simulink model "sampleModel2061"  (R2023a)
settings: Solver=VariableStepAuto  StartTime=0.0  StopTime=10.0  RelTol=1e-3
libraries: hdlsllib x5
settings Model: Creator=user1  LastModifiedBy=user1

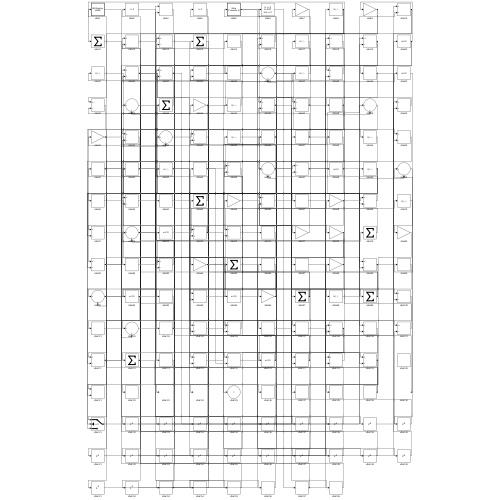
[thumbnail: Simulink's stored preview of the top-level diagram]
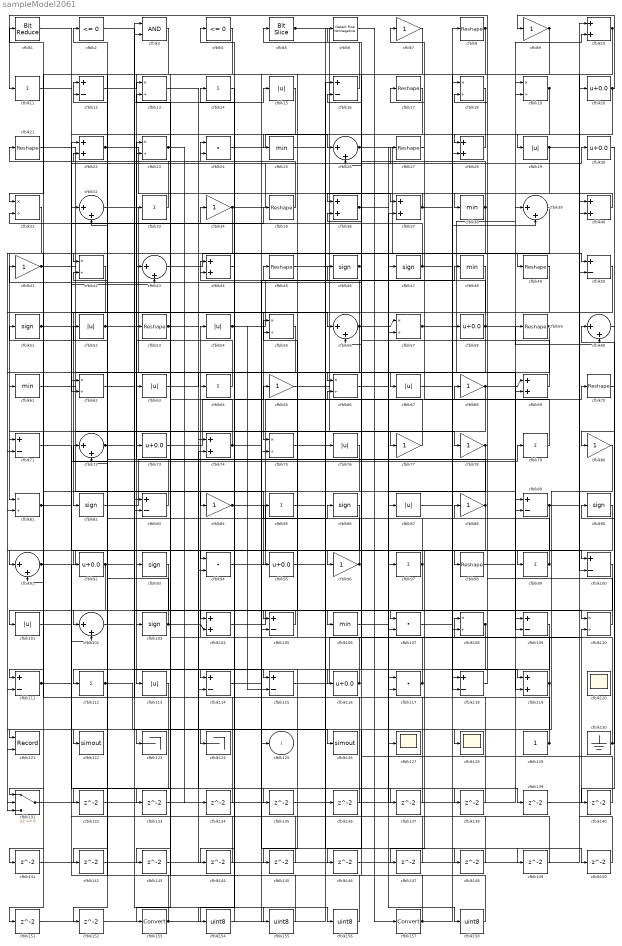
== system sampleModel2061 ==
  cfblk1 : hdlsllib/Logic and Bit Operations/Bit Reduce  mode=AND
  cfblk{10,22,28,36..37,40,44,69,74,104,119} (11 alike) : Sum
  cfblk{12,16,50,71,83,89,100,105,109,111,114..115,118} (13 alike) : Sum  Inputs=+-
  cfblk{15,29,52,54,63,67,76,87,101,113} (10 alike) : Abs  SaturateOnIntegerOverflow=off
  cfblk{26,32,39,43,56,60,72,91,102} (9 alike) : Sum  Inputs=|++
  cfblk{46..47,51,82,86,90,93,103} (8 alike) : Signum
  cfblk{25,38,48,61,106} (5 alike) : MinMax
  cfblk{24,94,107,117} (4 alike) : DotProduct  OutDataTypeStr=Inherit: Inherit via internal rule
  cfblk{13,18..19,23,31,42,55,57,62,66,75,81,108,110} (14 alike) : Product  Inputs=*/  RndMeth=Zero  SaturateOnIntegerOverflow=on
  cfblk{11,14,33,64,79,85,97,99,112} (9 alike) : Sum  Inputs=+
  cfblk{20,30,58,73,92,95,116} (7 alike) : Bias  Bias=0.0  SaturateOnIntegerOverflow=off
  cfblk120 : Scope
      settings: Floating=on
  cfblk121 : Record  FileSettingsInternal="{\"entries\":[{\"content\":{\"excelSettings\":{\"content\":{},\"type\":\"Streamout.ExcelSettings\"}},\"type\":\"Streamout.FileSettingStorage\",\"uuid\":\"\"}],\"packageUris\":[\"http:\\/\\/schema.mathworks.com\\/mf0\\/streamout_blocks\\/R2020a\"],\"version\":\"1.0\"}"  Layout=[1 1]  SignalsInternal="{\"entries\":[{\"content\":{\"signals\":[{\"content\":{\"blockPath\":[],\"dimensions\":[1],\"domain\":\"\",\"lineColor\":\"#a2142f\",\"plots\":[1],\"port\":1,\"signalID\":6369,\"signalName\":\"XY Graph:1\"},\"type\":\"RecordBlkView.Signal\",\"uuid\":\"\"},{\"content\":{\"blockPath\":[],\"dimensions\":[1],\"domain\":\"\",\"lineColor\":\"#139fff\",\"plots\":[1],\"port\":2,\"signalID\":6372,\"signalName\":\"XY Graph:2\"},\"type\":\"RecordBlkView.Signal\",\"uuid\":\"\"}]},\"type\":\"RecordBlkView.InputSignals\",\"uuid\":\"\"}],\"packageUris\":[\"http:\\/\\/schema.mathworks.com\\/mf0\\/streamout_blocks\\/R2020a\"],\"version\":\"1.0\"}"  VisualizationBindings="{\"xyplotplugin\":{\"info\":[{\"series\":[{\"bindingParametersList\":[{\"parameter\":\"X-Axis\",\"signalID\":6369,\"signalName\":\"XY Graph:1\"},{\"parameter\":\"Y-Axis\",\"signalID\":6372,\"signalName\":\"XY Graph:2\"}],\"seriesID\":44512}],\"subplotID\":1}]}}"  CompatibilityTag=XY  st=-1
  cfblk122 : ToWorkspace  VariableName=simout  SaveFormat=Timeseries  SampleTime=-1
  cfblk123 : Terminator
  cfblk124 : Terminator
  cfblk126 : ToWorkspace  VariableName=simout  SaveFormat=Timeseries  SampleTime=-1
  cfblk127 : Scope
  cfblk128 : Scope
  cfblk129 : Constant  SampleTime=-1
  cfblk130 : Ground
  cfblk131 : Switch  SaturateOnIntegerOverflow=off  InputSameDT=off
  cfblk{132..152} (21 alike) : Delay  SampleTime=1
  cfblk153 : DataTypeConversion  SaturateOnIntegerOverflow=off  RndMeth=Floor
  cfblk{154..156,158} (4 alike) : DataTypeConversion  OutDataTypeStr=uint8  SaturateOnIntegerOverflow=off  RndMeth=Floor
  cfblk157 : DataTypeConversion  SaturateOnIntegerOverflow=off  RndMeth=Floor
  cfblk{8,17,21,27,35,45,49,53,59,70,98} (11 alike) : Reshape
  cfblk2 : hdlsllib/Logic and Bit Operations/Compare To Zero  relop=<=  OutDataTypeStr=boolean
  cfblk3 : Logic  AllPortsSameDT=off  OutDataTypeStr=boolean
  cfblk{7,9,34,41,65,68,77..78,80,84,88,96} (12 alike) : Gain
  cfblk4 : hdlsllib/Logic and Bit Operations/Compare To Zero  relop=<=  OutDataTypeStr=boolean
  cfblk5 : hdlsllib/Logic and Bit Operations/Bit Slice  lidx=7  ridx=0
  cfblk6 : hdlsllib/Logic and Bit Operations/Detect Rise Nonnegative  vinit=0  OutDataTypeStr=boolean
  cfblk125 : Outport  VectorParamsAs1DForOutWhenUnconnected=off
  wires:
  cfblk76/1 -> cfblk113/1
  cfblk31/1 -> cfblk81/1
  cfblk8/1 -> cfblk103/1, cfblk105/1, cfblk105/2
  cfblk99/1 -> cfblk11/1, cfblk12/2
  cfblk5/1 -> cfblk77/1, cfblk148/1
  cfblk24/1 -> cfblk26/1
  cfblk42/1 -> cfblk82/1
  cfblk80/1 -> cfblk128/1
  cfblk94/1 -> cfblk70/1
  cfblk83/1 -> cfblk23/1
  cfblk17/1 -> cfblk102/1
  cfblk36/1 -> cfblk106/1, cfblk158/1
  cfblk81/1 -> cfblk79/1, cfblk35/1
  cfblk119/1 -> cfblk108/1, cfblk131/2, cfblk146/1
  cfblk116/1 -> cfblk54/1, cfblk43/1
  cfblk55/1 -> cfblk111/1
  cfblk56/1 -> cfblk57/1, cfblk14/1, cfblk100/1, cfblk91/2
  cfblk60/1 -> cfblk90/1
  cfblk58/1 -> cfblk45/1, cfblk60/2, cfblk71/2
  cfblk130/1 -> cfblk24/1, cfblk60/1
  cfblk6/1 -> cfblk157/1
  cfblk91/1 -> cfblk98/1, cfblk102/2
  cfblk15/1 -> cfblk63/1
  cfblk87/1 -> cfblk108/2
  cfblk79/1 -> cfblk17/1
  cfblk53/1 -> cfblk115/1, cfblk109/2
  cfblk49/1 -> cfblk101/1
  cfblk40/1 -> cfblk38/1
  cfblk78/1 -> cfblk141/1, cfblk142/1
  cfblk75/1 -> cfblk68/1
  cfblk52/1 -> cfblk109/1, cfblk114/2
  cfblk46/1 -> cfblk96/1, cfblk26/2
  cfblk21/1 -> cfblk95/1
  cfblk16/1 -> cfblk5/1
  cfblk112/1 -> cfblk126/1, cfblk12/1
  cfblk118/1 -> cfblk18/2
  cfblk32/1 -> cfblk89/1
  cfblk96/1 -> cfblk24/2, cfblk66/2
  cfblk27/1 -> cfblk7/1
  cfblk45/1 -> cfblk87/1
  cfblk117/1 -> cfblk64/1, cfblk55/2
  cfblk4/1 -> cfblk153/1
  cfblk23/1 -> cfblk123/1, cfblk134/1
  cfblk84/1 -> cfblk99/1, cfblk48/1
  cfblk18/1 -> cfblk28/1
  cfblk65/1 -> cfblk117/1
  cfblk69/1 -> cfblk41/1
  cfblk109/1 -> cfblk112/1
  cfblk1/1 -> cfblk56/1
  cfblk129/1 -> cfblk72/1, cfblk23/2
  cfblk11/1 -> cfblk32/1
  cfblk38/1 -> cfblk131/3, cfblk16/2, cfblk132/1
  cfblk39/1 -> cfblk122/1
  cfblk59/1 -> cfblk121/2, cfblk94/2, cfblk143/1
  cfblk26/1 -> cfblk50/1, cfblk89/2
  cfblk37/1 -> cfblk36/1, cfblk39/2
  cfblk34/1 -> cfblk27/1, cfblk94/1, cfblk61/1
  cfblk33/1 -> cfblk21/1
  cfblk19/1 -> cfblk29/1, cfblk83/2
  cfblk44/1 -> cfblk84/1
  cfblk71/1 -> cfblk93/1
  cfblk106/1 -> cfblk127/1
  cfblk62/1 -> cfblk107/1
  cfblk72/1 -> cfblk3/2, cfblk139/1
  cfblk97/1 -> cfblk92/1, cfblk85/1, cfblk55/1, cfblk151/1
  cfblk107/1 -> cfblk119/1
  cfblk100/1 -> cfblk107/2
  cfblk25/1 -> cfblk37/1
  cfblk89/1 -> cfblk20/1, cfblk147/1
  cfblk67/1 -> cfblk119/2
  cfblk29/1 -> cfblk50/2, cfblk116/1
  cfblk63/1 -> cfblk67/1
  cfblk115/1 -> cfblk40/1
  cfblk114/1 -> cfblk86/1
  cfblk86/1 -> cfblk111/2
  cfblk108/1 -> cfblk144/1, cfblk145/1
  cfblk64/1 -> cfblk33/1
  cfblk57/1 -> cfblk19/2, cfblk69/2
  cfblk50/1 -> cfblk75/1
  cfblk54/1 -> cfblk46/1, cfblk115/2
  cfblk68/1 -> cfblk69/1, cfblk124/1
  cfblk73/1 -> cfblk65/1
  cfblk92/1 -> cfblk15/1, cfblk121/1
  cfblk98/1 -> cfblk10/2
  cfblk41/1 -> cfblk125/1, cfblk91/1
  cfblk48/1 -> cfblk81/2
  cfblk105/1 -> cfblk104/1
  cfblk111/1 -> cfblk34/1, cfblk30/1
  cfblk93/1 -> cfblk131/1
  cfblk103/1 -> cfblk104/2, cfblk42/2
  cfblk47/1 -> cfblk8/1, cfblk31/2
  cfblk104/1 -> cfblk110/1
  cfblk82/1 -> cfblk59/1
  cfblk43/1 -> cfblk49/1
  cfblk61/1 -> cfblk78/1
  cfblk88/1 -> cfblk51/1, cfblk117/2
  cfblk131/1 -> cfblk39/1
  cfblk3/1 -> cfblk31/1
  cfblk66/1 -> cfblk47/1
  cfblk12/1 -> cfblk13/1
  cfblk7/1 -> cfblk72/2
  cfblk9/1 -> cfblk66/1, cfblk133/1
  cfblk35/1 -> cfblk13/2
  cfblk30/1 -> cfblk80/1
  cfblk90/1 -> cfblk114/1
  cfblk20/1 -> cfblk9/1, cfblk42/1, cfblk62/2
  cfblk74/1 -> cfblk71/1, cfblk53/1, cfblk149/1
  cfblk51/1 -> cfblk83/1, cfblk43/2
  cfblk10/1 -> cfblk118/2, cfblk100/2
  cfblk22/1 -> cfblk74/1, cfblk97/1
  cfblk110/1 -> cfblk88/1
  cfblk28/1 -> cfblk25/1
  cfblk77/1 -> cfblk44/1
  cfblk132/1 -> cfblk19/1
  cfblk133/1 -> cfblk57/2
  cfblk134/1 -> cfblk1/1
  cfblk101/1 -> cfblk135/1
  cfblk135/1 -> cfblk37/2
  cfblk95/1 -> cfblk136/1
  cfblk136/1 -> cfblk16/1
  cfblk102/1 -> cfblk137/1
  cfblk137/1 -> cfblk3/1
  cfblk13/1 -> cfblk138/1
  cfblk138/1 -> cfblk118/1
  cfblk139/1 -> cfblk110/2
  cfblk70/1 -> cfblk140/1
  cfblk140/1 -> cfblk56/2
  cfblk141/1 -> cfblk18/1
  cfblk142/1 -> cfblk74/2
  cfblk143/1 -> cfblk28/2
  cfblk144/1 -> cfblk62/1
  cfblk145/1 -> cfblk32/2
  cfblk146/1 -> cfblk40/2
  cfblk147/1 -> cfblk44/2
  cfblk148/1 -> cfblk22/2
  cfblk149/1 -> cfblk36/2
  cfblk85/1 -> cfblk150/1
  cfblk150/1 -> cfblk10/1
  cfblk151/1 -> cfblk75/2
  cfblk113/1 -> cfblk152/1
  cfblk152/1 -> cfblk76/1
  cfblk153/1 -> cfblk52/1, cfblk156/1
  cfblk14/1 -> cfblk154/1
  cfblk154/1 -> cfblk4/1
  cfblk2/1 -> cfblk155/1
  cfblk155/1 -> cfblk73/1
  cfblk156/1 -> cfblk2/1
  cfblk157/1 -> cfblk58/1, cfblk22/1
  cfblk158/1 -> cfblk6/1
